simulink model "HW2_Q.1"  (R2017b)
settings: Solver=VariableStepAuto  StartTime=-5  StopTime=15  RelTol=1e-3
settings Model: Creator=ali  LastModifiedBy=ali

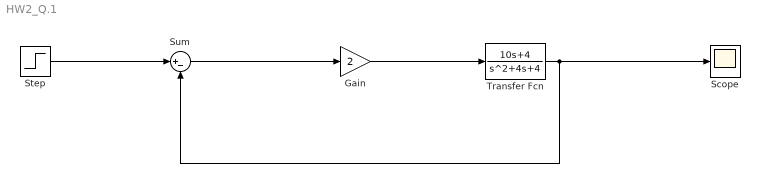
== system HW2_Q.1 ==
  Gain : Gain  Gain=2
  Scope : Scope
  Step : Step  Time=0  SampleTime=0
  Sum : Sum  Inputs=|+-
  Transfer Fcn : TransferFcn  Numerator=[0 10 4]  Denominator=[1 4 4]
  wires:
  Step/1 -> Sum/1
  Sum/1 -> Gain/1
  Gain/1 -> Transfer Fcn/1
  Transfer Fcn/1 -> Sum/2, Scope/1
